simulink model "smm_with_grf_tilting_2d"  (R2014b)
settings: Solver=FixedStepDiscrete  StartTime=0.0  StopTime=inf  FixedStep=sample_time  RelTol=1e-3
undefined symbols (not defined in the file or in its folder): A_lpf_dtau, A_lpf_leg_spring, alpha_apex, alpha_max, alpha_min, B1_lpf_dtau, B1_lpf_leg_spring, B2_lpf_dtau, B2_lpf_leg_spring, boom_mount_angle, boom_pelvis_offset_angle, c_energy, contact_threshold, control_start_time, d_y_boom_com_offset, d_y_boom_hip_offset, d_y_com, desired_torso_angle, dx_avg_desired, enable_torso_wave, fcut_contact, ff_energy_l, ff_energy_r, g, g_reduced, h_boom, HIP_MTR_MAX_CONT_TORQUE, i_robot, initial_com_height, initial_dx, j_leg, j_motor, j_rotor, j_segments, k0_virtual, k_placement, k_sea, kd_lateral, kd_motor, kd_torso, kp_lateral, kp_motor, kp_raibert, kp_torso, l0_leg, l0_min_flight_time, l0_virtual, l0_virtual_raibert, l_boom_projected, l_max, l_retract_delta, l_retract_swing_max, l_retract_swing_min, l_seg, l_yaw_center_to_pelvis, lambda1, lambda2, lateral_offset, lateral_target_angle_left, lateral_target_angle_right ... (+40)
libraries: simulink x24, slrtlib x4, simulink_extras x2
(part 4 of 4)

== matlab function smm_with_grf_tilting_2d/Control/Behavior Control/Secondary Leg Behavior/Virtual Leg Trajectory Towards Alpha Apex Target ==
  data: start input; t_system input; l_leg output; dl_leg output; ddl_leg output; phi output; dphi output; ddphi output; alpha_apex parameter; theta input; l_measured input; dl_measured input; phi_measured input; dphi_measured input; d_y_com parameter; l0_virtual parameter
%% Create a trajectory between starting position/velocity and some alpha
% The goal is to move the system towards the alpha target at apex.
function [l_leg, dl_leg, ddl_leg, phi, dphi, ddphi] = fcn(start, t_system, alpha_apex, theta, l_measured, dl_measured, phi_measured, dphi_measured, d_y_com, l0_virtual)
    % Should the target be less than apex position? midpoint?
    [l_apex, dl_apex, ~, phi_apex, dphi_apex, ~] = AlphaTargetToVirtualLeg2D(alpha_apex, 0, 0, theta, 0, 0, d_y_com, l0_virtual);
    
    % Force retraction when secondary leg
    l_apex = 0.8;
    dl_apex = 0;
    
    persistent t_start l_start phi_start dl_start dphi_start;
    if isempty(t_start)
        t_start = t_system;
        l_start = l_measured;
        dl_start = dl_measured;
        phi_start = phi_measured;
        dphi_start = dphi_measured;
    end
    if start %|| (t_system - t_start) > 0.030
        t_start = t_system;
        l_start = l_measured;
        dl_start = dl_measured;
        phi_start = phi_measured;
        dphi_start = dphi_measured;
    end
    

    time_to_takeoff = 0.350;  % Overestimate, How to approximate this?
    t = t_system - t_start;
    t = min(time_to_takeoff, t);
    
    % Virtual Leg Length
    [a0, a1, a2, a3] = ThirdOrderTrajectory(l_start, dl_start, l_apex, dl_apex, time_to_takeoff);
    l_leg = a3*t^3 + a2*t^2 + a1*t + a0;
    dl_leg = 3*a3*t^2 + 2*a2*t + a1;
    ddl_leg = 6*a3*t + 2*a2;
    
    % Virtual Leg Angle
    [a0, a1, a2, a3] = ThirdOrderTrajectory(phi_start, dphi_start, phi_apex, dphi_apex, time_to_takeoff);
    phi = a3*t^3 + a2*t^2 + a1*t + a0;
    dphi = 3*a3*t^2 + 2*a2*t + a1;
    ddphi = 6*a3*t + 2*a2;
end

== matlab function smm_with_grf_tilting_2d/Control/Behavior Control/Secondary Leg Behavior/Virtual Leg to Four Bar ==
  data: l_leg input; dl_leg input; ddl_leg input; phi input; dphi input; ddphi input; back output; dback output; ddback output; front output; dfront output; ddfront output
function [back, dback, ddback, front, dfront, ddfront] = VirtualLegToFourBar(l_leg, dl_leg, ddl_leg, phi, dphi, ddphi)
    [back, dback, ddback, front, dfront, ddfront] = VirtualLegToFourBar(l_leg, dl_leg, ddl_leg, phi, dphi, ddphi);
end

== matlab function smm_with_grf_tilting_2d/Control/Behavior Control/Primary Leg Behavior/SMM 01/Primary Swing Phase/Leg Trajectory Generator (Level Ground)/Alpha Target to Leg Length and Leg Angle ==
  data: alpha_v input; dalpha_v input; ddalpha_v input; theta input; dtheta input; l output; dl output; ddl output; phi output; d_y_com parameter; l0_virtual parameter; dphi output; ddphi output
function [l, dl, ddl, phi, dphi, ddphi] = fcn(alpha_v, dalpha_v, ddalpha_v, theta, dtheta, d_y_com, l0_virtual)
    [l, dl, ddl, phi, dphi, ddphi] = AlphaTargetToVirtualLeg2D(alpha_v, dalpha_v, ddalpha_v, theta, dtheta, 0, d_y_com, l0_virtual);
end

== matlab function smm_with_grf_tilting_2d/Control/Behavior Control/Primary Leg Behavior/SMM 01/Primary Swing Phase/Leg Trajectory Generator (Level Ground)/Retracted Leg Trajectory ==
  data: start input; t_system input; t_apex input; l_apex input; dl_apex input; phi_apex input; dphi_apex input; l_measured input; dl_measured input; phi_measured input; l output; dl output; ddl output; phi output; dphi output; ddphi output; dphi_measured input
%% Generates a dynamically feasible trajectory for swinging the virtual leg between two points.
% Constrains to starting/ending positions and velocities.
% Minimizes torque squared
% May want to generate the trajectory in fourbar coordinates instead.
function [l, dl, ddl, phi, dphi, ddphi] = fcn(start, t_system, t_apex, l_apex, dl_apex, phi_apex, dphi_apex, l_measured, dl_measured, phi_measured, dphi_measured)

    persistent t_start l_start phi_start dl_start dphi_start;
    if isempty(t_start) || start
        t_start = t_system;
        l_start = l_measured;
        dl_start = dl_measured;
        phi_start = phi_measured;
        dphi_start = dphi_measured;
    end
    
    t = t_system - t_start;
    time_to_apex = 0.95*2*(t_apex - t_start);
    t = min(time_to_apex, t);

    % Virtual Leg Length
    [a0, a1, a2, a3] = ThirdOrderTrajectory(l_start, dl_start, l_apex, dl_apex, time_to_apex);
    l = a3*t^3 + a2*t^2 + a1*t + a0;
    dl = 3*a3*t^2 + 2*a2*t + a1;
    ddl = 6*a3*t + 2*a2;
    
    % Virtual Leg Angle
    [a0, a1, a2, a3] = ThirdOrderTrajectory(phi_start, dphi_start, phi_apex, dphi_apex, time_to_apex);
    phi = a3*t^3 + a2*t^2 + a1*t + a0;
    dphi = 3*a3*t^2 + 2*a2*t + a1;
    ddphi = 6*a3*t + 2*a2;

end

== matlab function smm_with_grf_tilting_2d/Control/Behavior Control/Primary Leg Behavior/SMM 01/Primary Swing Phase/Avoid Hitting Mechanical Limits1 ==
  data: back_cmd output; front_cmd output; dback_cmd output; dfront_cmd output; ddback_cmd output; ddfront_cmd output; back_desired input; dback_desired input; ddback_desired input; front_desired input; dfront_desired input; ddfront_desired input; min_front_bar_angle parameter; max_front_bar_angle parameter; min_back_bar_angle parameter; max_back_bar_angle parameter
%% Avoid joint limits by ensuring we don't command velocities/accelerations that would push us into them when we are close to them.
function [back_cmd, front_cmd, dback_cmd, dfront_cmd, ddback_cmd, ddfront_cmd] ...
    = AvoidFourbarLimits(back_desired,dback_desired, ddback_desired, ...
          front_desired, dfront_desired, ddfront_desired, ...
          min_front_bar_angle, max_front_bar_angle, min_back_bar_angle, max_back_bar_angle)
    [back_cmd, front_cmd, dback_cmd, dfront_cmd, ddback_cmd, ddfront_cmd] = AvoidFourbarLimits(back_desired,dback_desired, ddback_desired, front_desired, dfront_desired, ddfront_desired, min_front_bar_angle, max_front_bar_angle, min_back_bar_angle, max_back_bar_angle);
end

== matlab function smm_with_grf_tilting_2d/Control/Behavior Control/Primary Secondary Leg Swap/ToggleRightLeftLeg ==
  data: toggle input boolean; right_left output double; previous_right_left input double
function right_left = ToggleRightLeftLeg(toggle, previous_right_left)
    
    if toggle
        right_left = -previous_right_left + 1;
    else
        right_left = previous_right_left;
    end

end

== matlab function smm_with_grf_tilting_2d/Control/Behavior Control/Lateral Control ==
  data: tau_r output size=1; qLateralR input; dqLateralR input; qLateralL input; dqLateralL input; F_leg_R input; F_leg_L input; L_leg_R input; L_leg_L input; lateral_transition_force parameter; lateral_target_angle_right parameter; lateral_target_angle_left parameter; boom_mount_angle parameter; boom_pelvis_offset_angle parameter; l_yaw_center_to_pelvis parameter; m_leg_motor parameter; g parameter; lateral_offset parameter; tau_l output size=1; kp_lateral parameter; kd_lateral parameter; minimum_lateral_angle parameter; maximum_lateral_angle parameter; HIP_MTR_MAX_CONT_TORQUE parameter
function [tau_r, tau_l] = LateralBoomControl(qLateralR, dqLateralR, qLateralL, dqLateralL, F_leg_R, F_leg_L, L_leg_R, L_leg_L, lateral_transition_force, lateral_target_angle_right, lateral_target_angle_left, boom_mount_angle, boom_pelvis_offset_angle, l_yaw_center_to_pelvis, m_leg_motor, g, lateral_offset, kp_lateral, kd_lateral, minimum_lateral_angle, maximum_lateral_angle, HIP_MTR_MAX_CONT_TORQUE)

    gravity_compensation = m_leg_motor*g*lateral_offset;
    if (F_leg_R < lateral_transition_force && F_leg_L < lateral_transition_force), gravity_compensation = 0; end % freefall
    
    % Right Leg
    desired = saturate([lateral_target_angle_right, 0],minimum_lateral_angle,maximum_lateral_angle);
    measured = [qLateralR, dqLateralR];
    tau_r = [kp_lateral, kd_lateral] * (desired-measured)' + gravity_compensation;
    tau_r = max(min(HIP_MTR_MAX_CONT_TORQUE, tau_r),-HIP_MTR_MAX_CONT_TORQUE);
    
    if (F_leg_R >= lateral_transition_force)
        angle = qLateralR - boom_pelvis_offset_angle + boom_mount_angle;
        J =   (L_leg_R - l_yaw_center_to_pelvis*sin(angle)) ./ (L_leg_R.*l_yaw_center_to_pelvis.*cos(angle) - l_yaw_center_to_pelvis*lateral_offset*sin(angle));    
        tau_r = -F_leg_R*(J - lateral_offset) + gravity_compensation;
    end
    
    % Left Leg
    desired = saturate([lateral_target_angle_left, 0],minimum_lateral_angle,maximum_lateral_angle);
    measured = [qLateralL, dqLateralL];
    tau_l = [kp_lateral, kd_lateral] * (desired-measured)' + gravity_compensation;
    tau_l = max(min(HIP_MTR_MAX_CONT_TORQUE, tau_l),-HIP_MTR_MAX_CONT_TORQUE);
    
    if (F_leg_L >= lateral_transition_force)
        angle = qLateralL + boom_pelvis_offset_angle - boom_mount_angle;
        J =  -(L_leg_L + l_yaw_center_to_pelvis*sin(angle)) ./ (L_leg_L.*l_yaw_center_to_pelvis.*cos(angle) - l_yaw_center_to_pelvis*lateral_offset*sin(angle));  
        tau_l = F_leg_L*(J - lateral_offset) + gravity_compensation;  
    end
    
    % Stance
%     if ~escape
%         if ~placement && right_or_left
%             angle = qLateralR - boom_pelvis_offset_angle + boom_mount_angle;
%             J =   (l_leg - l_yaw_center_to_pelvis*sin(angle)) ./ (l_leg.*l_yaw_center_to_pelvis.*cos(angle) - l_yaw_center_to_pelvis*lateral_offset*sin(angle));    
%             tau_r = -F_leg*(J - lateral_offset) + gravity_compensation; % + lateral_offset ???  -F*(J+r) + g       F*(J-r) + g
%         elseif ~placement && ~right_or_left
%             angle = qLateralL + boom_pelvis_offset_angle - boom_mount_angle;
%             J =  -(l_leg + l_yaw_center_to_pelvis*sin(angle)) ./ (l_leg.*l_yaw_center_to_pelvis.*cos(angle) - l_yaw_center_to_pelvis*lateral_offset*sin(angle));  
%             tau_l = F_leg*(J - lateral_offset) + gravity_compensation;
%         end
%     end
end

function [desired_saturated] = saturate(desired, minimum_lateral_angle, maximum_lateral_angle)
    desired_saturated = desired;
    if desired(1) < minimum_lateral_angle
        desired_saturated = [minimum_lateral_angle, 0];
    elseif desired(1) > maximum_lateral_angle
        desired_saturated = [maximum_lateral_angle, 0];    
    end
end

== matlab function smm_with_grf_tilting_2d/Control/Behavior Control/Primary Leg Behavior/Raibert Hopping/Inverse Dynamics Virtual Spring/target_GRF_inverse_dynamics ==
  data: z output; k_virtual input; l_virtual input; theta input; phi input; l_leg input; w input; tau_rotor_f input; tau_rotor_b input; d_y_com parameter; l_virtual_rest input; LEG_MTR_GEAR_RATIO parameter; g parameter; j_leg parameter; j_rotor parameter; i_robot parameter; m_total_real parameter; m_boom parameter; m_leg parameter; GRFx output; GRFy output; kp_torso parameter; kd_torso parameter; desired_torso_angle input; GRF_angle output; max_GRF_angle parameter
%% Inverse dynamics
% Inputs:  gamma, dgamma, theta, dtheta,  GRFx_des, GRFy_des
% Outputs: ddx,   ddy,    ddl,   ddgamma, ddtheta,  tau_sf,  tau_sb
function [z, GRFx, GRFy, GRF_angle]  = fcn(k_virtual, l_virtual, theta, phi, l_leg, w,...
                  tau_rotor_f, tau_rotor_b, ...
                  d_y_com, l_virtual_rest, LEG_MTR_GEAR_RATIO, g,...
                  j_leg, j_rotor, i_robot, ...
                  m_total_real, m_boom, m_leg, ...
                  kp_torso, kd_torso, desired_torso_angle, max_GRF_angle)

              
              
    % Parameters
    m      = m_total_real;    % mass of system + boom
    Il     = j_leg;             % inertia of leg
    Ir     = j_rotor;           % inertia of rotor
    It     = i_robot;           % inertia of system
    d      = d_y_com;             % distance from hip to system COM
    g1     = phi(1)+theta(1);   % global leg angle (after spring)
    dg1    = phi(2)+theta(2);
    th     = theta(1);          % global torso angle   
    dth    = theta(2);
    t_rf   = tau_rotor_f;       % torque applied at front rotor 
    t_rb   = tau_rotor_b;       % torque applied at back rotor
    N      = -LEG_MTR_GEAR_RATIO;
    l      = l_leg(1);          % leg length
    dl     = l_leg(2);
    lv     = l_virtual(1);      % virtual spring length
    dx     = -l*dg1*cos(g1)+dth*cos(th);
    dy     = l*dg1*sin(g1)-dth*sin(th);
    
    
    
    % Target GRFs
    delta_lv = l_virtual_rest -  lv;
    GRF = k_virtual*delta_lv* ...
                        [(d*sin(th)-l*sin(g1))/lv; ...
                         (d*cos(th)-l*cos(g1))/lv];
    GRF_angle = atan2(GRF(2),GRF(1));
                     
                     
                     
    % Trunk posture correction 
    % l_leg cross GRF = I_robot * ddtheta
    F_reg = 1; % prevent division by zero
    ddth_desired = kp_torso*(desired_torso_angle - th) - kd_torso*dth; % PD law
    sine_ratio = It*ddth_desired / (lv*(norm(GRF) + F_reg));
    max_angle = 20*pi/180;
    sine_ratio = min(sin(max_angle), max(-sin(max_angle), sine_ratio));  % saturate rotation angle
    GRF_rotation = asin(sine_ratio);
    GRF_full_angle = GRF_rotation + GRF_angle; % saturate GRF angle
    if GRF_full_angle > (pi-max_GRF_angle)
        GRF_rotation = (pi-max_GRF_angle) - GRF_angle;
    elseif GRF_full_angle < max_GRF_angle
        GRF_rotation = max_GRF_angle - GRF_angle;  
    end
    R = [cos(GRF_rotation)  -sin(GRF_rotation); sin(GRF_rotation) cos(GRF_rotation)];
    GRF_target = R*GRF; % rotate GRF CCW
    GRFx = GRF_target(1);
    GRFy = GRF_target(2);
    GRF_angle = atan2(GRFy,GRFx);
    
    
    
    
    % Stance dynamics (P z = [h; -dJ*dq] + [J zeros(2,2)]^T F)
    %     J  = [1  0  sin(g1)     l*cos(g1)   -d*cos(th);
    %           0  1  cos(g1)    -l*sin(g1)    d*sin(th)];
    %       
    %     dJ = [0  0   dg1*cos(g1)    (-l*dg1*sin(g1)+dl*cos(g1))  d*dth*sin(th);
    %           0  0  -dg1*sin(g1)    (-1*dg1*cos(g1)-dl*sin(g1))  d*dth*cos(th)];
    % 
    %     dq  = [dx  dy  dl  dg1  dth ]';
    %       
    %     M = [m  0   0       0    0; 
    %          0  m   0       0    0;
    %          0  0   m_leg   0    0;   
    %          0  0   0       Il   0;  
    %          0  0   0       0    It];  
    %     
    %     h = [0; -m*g_reduced; 0; 0; (-t_rf-t_rb)];
    % 
    %     S = [ 0         0;
    %           0         0;
    %           1/w      -1/w;
    %           1         1;
    %          -(N-1)/N  -(N-1)/N];
    % 
    %     F = [GRFx GRFy]';
    %     
    %     P = [M              -S;       
    %          J               zeros(2,2)];
    
    % Solving for z:    
    %     ddq = [ddx ddy ddl ddg1 ddth]';
    %     z = [ddq; t_sf; t_sb];
    %     z = P\([h; -dJ*dq] + [J zeros(2,2)]'*F);
    
    z =  [GRFx/m;
         (GRFy - g*m)/m;
        -(Il*d*dg1^2*m*cos(g1 - th) - 2*GRFx*Il*d*sin(th) - 2*Il*d^2*dth^2*m - GRFy*d*l^2*m*cos(th) - GRFx*d*l^2*m*sin(th) - 2*GRFy*Il*d*cos(th) + 2*GRFy*It*N*l*cos(g1) + 2*GRFy*Il*N*d*cos(th) + 2*GRFx*It*N*l*sin(g1) + 2*GRFx*Il*N*d*sin(th) - It*N*dg1^2*l*m + GRFy*d*l^2*m*cos(2*g1 - th) + GRFx*d*l^2*m*sin(2*g1 - th) + 2*Il*d*g*m*cos(th) + Il*d*dg1^2*m*cos(g1 + th) + 2*Il*N*d^2*dth^2*m - It*N*dg1^2*l^2*m - 2*It*N*g*l*m*cos(g1) - 2*Il*N*d*g*m*cos(th) + It*N*dg1^2*l^2*m*cos(2*g1) - Il*N*d*dg1^2*m*cos(g1 + th) - Il*d*dg1^2*l*m*cos(g1 + th) + 4*Il*d*dg1*dl*m*sin(g1 - th) + GRFy*N*d^2*l*m*cos(g1) + GRFy*N*d*l^2*m*cos(th) + GRFx*N*d^2*l*m*sin(g1) + 2*N*d*l*m*t_rb*sin(g1 - th) + 2*N*d*l*m*t_rf*sin(g1 - th) + GRFx*N*d*l^2*m*sin(th) - Il*N*d*dg1^2*m*cos(g1 - th) - GRFy*N*d^2*l*m*cos(g1 - 2*th) + GRFx*N*d^2*l*m*sin(g1 - 2*th) + Il*d*dg1^2*l*m*cos(g1 - th) - It*N*dg1^2*l*m*cos(2*g1) - GRFy*N*d*l^2*m*cos(2*g1 - th) - GRFx*N*d*l^2*m*sin(2*g1 - th) + Il*N*d*dg1^2*l*m*cos(g1 + th) - 4*Il*N*d*dg1*dl*m*sin(g1 - th) - Il*N*d*dg1^2*l*m*cos(g1 - th) + 2*It*N*d*dth^2*l*m*cos(g1 - th))/(2*m*(It*N*l - Il*d*cos(g1 - th) + Il*N*d*cos(g1 - th)));
        -(2*GRFx*It*N*cos(g1) - 2*GRFy*It*N*sin(g1) + GRFx*N*d^2*m*cos(g1 - 2*th) + 4*It*N*dg1*dl*m + GRFy*N*d^2*m*sin(g1 - 2*th) + GRFx*d*l*m*cos(2*g1 - th) - GRFy*d*l*m*sin(2*g1 - th) + It*N*dg1^2*m*sin(2*g1) + 2*It*N*g*m*sin(g1) + GRFx*d*l*m*cos(th) - GRFy*d*l*m*sin(th) + GRFx*N*d^2*m*cos(g1) + 2*N*d*m*t_rb*cos(g1 - th) + 2*N*d*m*t_rf*cos(g1 - th) - GRFy*N*d^2*m*sin(g1) - GRFx*N*d*l*m*cos(th) + GRFy*N*d*l*m*sin(th) - GRFx*N*d*l*m*cos(2*g1 - th) - 2*It*N*d*dth^2*m*sin(g1 - th) + GRFy*N*d*l*m*sin(2*g1 - th) - It*N*dg1^2*l*m*sin(2*g1))/(2*m*(It*N*l - Il*d*cos(g1 - th) + Il*N*d*cos(g1 - th)));
        -(GRFx*Il*cos(g1) - GRFy*Il*sin(g1) - GRFx*Il*N*cos(g1) + (Il*dg1^2*m*sin(2*g1))/2 + GRFy*Il*N*sin(g1) + Il*g*m*sin(g1) + GRFx*l^2*m*cos(g1) - GRFy*l^2*m*sin(g1) + 2*Il*dg1*dl*m + N*l*m*t_rb + N*l*m*t_rf + GRFy*N*l^2*m*sin(g1) - 2*Il*N*dg1*dl*m - Il*d*dth^2*m*sin(g1 - th) - (Il*N*dg1^2*m*sin(2*g1))/2 - (Il*dg1^2*l*m*sin(2*g1))/2 - Il*N*g*m*sin(g1) - GRFx*N*l^2*m*cos(g1) + GRFx*N*d*l*m*cos(th) - GRFy*N*d*l*m*sin(th) + Il*N*d*dth^2*m*sin(g1 - th) + (Il*N*dg1^2*l*m*sin(2*g1))/2)/(m*(It*N*l - Il*d*cos(g1 - th) + Il*N*d*cos(g1 - th)));
        -(2*GRFx*Il*It*N*cos(g1) - 2*GRFy*Il*It*N*sin(g1) - GRFy*Il*d*m*w*cos(th) - 2*GRFy*Il*d*m_leg*w*cos(th) - GRFx*Il*d*m*w*sin(th) - 2*GRFx*Il*d*m_leg*w*sin(th) + GRFx*Il*N*d^2*m*cos(g1) + 2*Il*N*d*m*t_rb*cos(g1 - th) + 2*Il*N*d*m*t_rf*cos(g1 - th) + 2*GRFx*It*N*l^2*m*cos(g1) - GRFy*Il*N*d^2*m*sin(g1) - 2*GRFy*It*N*l^2*m*sin(g1) + GRFx*Il*N*d^2*m*cos(g1 - 2*th) + 4*Il*It*N*dg1*dl*m + GRFy*Il*N*d^2*m*sin(g1 - 2*th) - 2*Il*d^2*dth^2*m*m_leg*w - GRFy*Il*d*m*w*cos(2*g1 - th) - GRFx*Il*d*m*w*sin(2*g1 - th) + Il*It*N*dg1^2*m*sin(2*g1) + 2*Il*It*N*g*m*sin(g1) - GRFx*d*l^2*m*m_leg*w*sin(th) - Il*It*N*dg1^2*l*m*sin(2*g1) + Il*d*dg1^2*m*m_leg*w*cos(g1 - th) + 2*GRFy*It*N*l*m*w*cos(g1) + 2*GRFy*It*N*l*m_leg*w*cos(g1) + GRFy*Il*N*d*m*w*cos(th) + 2*GRFy*Il*N*d*m_leg*w*cos(th) + 2*GRFx*It*N*l*m*w*sin(g1) + 2*GRFx*It*N*l*m_leg*w*sin(g1) + GRFx*Il*N*d*m*w*sin(th) + 2*GRFx*Il*N*d*m_leg*w*sin(th) - It*N*dg1^2*l*m*m_leg*w + GRFy*d*l^2*m*m_leg*w*cos(2*g1 - th) + GRFx*d*l^2*m*m_leg*w*sin(2*g1 - th) + 2*Il*d*g*m*m_leg*w*cos(th) + Il*d*dg1^2*m*m_leg*w*cos(g1 + th) + 2*Il*N*d^2*dth^2*m*m_leg*w - It*N*dg1^2*l^2*m*m_leg*w - 2*Il*It*N*d*dth^2*m*sin(g1 - th) + GRFy*Il*N*d*m*w*cos(2*g1 - th) + GRFx*Il*N*d*m*w*sin(2*g1 - th) - GRFy*d*l^2*m*m_leg*w*cos(th) + It*N*dg1^2*l^2*m*m_leg*w*cos(2*g1) - Il*N*d*dg1^2*m*m_leg*w*cos(g1 + th) - Il*d*dg1^2*l*m*m_leg*w*cos(g1 + th) + 4*Il*d*dg1*dl*m*m_leg*w*sin(g1 - th) + GRFy*N*d^2*l*m*m_leg*w*cos(g1) + GRFy*N*d*l^2*m*m_leg*w*cos(th) + GRFx*N*d^2*l*m*m_leg*w*sin(g1) + 2*N*d*l*m*m_leg*t_rb*w*sin(g1 - th) + 2*N*d*l*m*m_leg*t_rf*w*sin(g1 - th) + GRFx*N*d*l^2*m*m_leg*w*sin(th) - Il*N*d*dg1^2*m*m_leg*w*cos(g1 - th) - GRFy*N*d^2*l*m*m_leg*w*cos(g1 - 2*th) + GRFx*N*d^2*l*m*m_leg*w*sin(g1 - 2*th) + Il*d*dg1^2*l*m*m_leg*w*cos(g1 - th) - It*N*dg1^2*l*m*m_leg*w*cos(2*g1) - GRFy*N*d*l^2*m*m_leg*w*cos(2*g1 - th) - GRFx*N*d*l^2*m*m_leg*w*sin(2*g1 - th) - 2*It*N*g*l*m*m_leg*w*cos(g1) - 2*Il*N*d*g*m*m_leg*w*cos(th) + Il*N*d*dg1^2*l*m*m_leg*w*cos(g1 + th) - 4*Il*N*d*dg1*dl*m*m_leg*w*sin(g1 - th) - Il*N*d*dg1^2*l*m*m_leg*w*cos(g1 - th) + 2*It*N*d*dth^2*l*m*m_leg*w*cos(g1 - th))/(4*m*(It*N*l - Il*d*cos(g1 - th) + Il*N*d*cos(g1 - th)));
         (2*GRFy*Il*It*N*sin(g1) - 2*GRFx*Il*It*N*cos(g1) - GRFy*Il*d*m*w*cos(th) - 2*GRFy*Il*d*m_leg*w*cos(th) - GRFx*Il*d*m*w*sin(th) - 2*GRFx*Il*d*m_leg*w*sin(th) - GRFx*Il*N*d^2*m*cos(g1) - 2*Il*N*d*m*t_rb*cos(g1 - th) - 2*Il*N*d*m*t_rf*cos(g1 - th) - 2*GRFx*It*N*l^2*m*cos(g1) + GRFy*Il*N*d^2*m*sin(g1) + 2*GRFy*It*N*l^2*m*sin(g1) - GRFx*Il*N*d^2*m*cos(g1 - 2*th) - 4*Il*It*N*dg1*dl*m - GRFy*Il*N*d^2*m*sin(g1 - 2*th) - 2*Il*d^2*dth^2*m*m_leg*w - GRFy*Il*d*m*w*cos(2*g1 - th) - GRFx*Il*d*m*w*sin(2*g1 - th) - Il*It*N*dg1^2*m*sin(2*g1) - 2*Il*It*N*g*m*sin(g1) - GRFx*d*l^2*m*m_leg*w*sin(th) + Il*It*N*dg1^2*l*m*sin(2*g1) + Il*d*dg1^2*m*m_leg*w*cos(g1 - th) + 2*GRFy*It*N*l*m*w*cos(g1) + 2*GRFy*It*N*l*m_leg*w*cos(g1) + GRFy*Il*N*d*m*w*cos(th) + 2*GRFy*Il*N*d*m_leg*w*cos(th) + 2*GRFx*It*N*l*m*w*sin(g1) + 2*GRFx*It*N*l*m_leg*w*sin(g1) + GRFx*Il*N*d*m*w*sin(th) + 2*GRFx*Il*N*d*m_leg*w*sin(th) - It*N*dg1^2*l*m*m_leg*w + GRFy*d*l^2*m*m_leg*w*cos(2*g1 - th) + GRFx*d*l^2*m*m_leg*w*sin(2*g1 - th) + 2*Il*d*g*m*m_leg*w*cos(th) + Il*d*dg1^2*m*m_leg*w*cos(g1 + th) + 2*Il*N*d^2*dth^2*m*m_leg*w - It*N*dg1^2*l^2*m*m_leg*w + 2*Il*It*N*d*dth^2*m*sin(g1 - th) + GRFy*Il*N*d*m*w*cos(2*g1 - th) + GRFx*Il*N*d*m*w*sin(2*g1 - th) - GRFy*d*l^2*m*m_leg*w*cos(th) + It*N*dg1^2*l^2*m*m_leg*w*cos(2*g1) - Il*N*d*dg1^2*m*m_leg*w*cos(g1 + th) - Il*d*dg1^2*l*m*m_leg*w*cos(g1 + th) + 4*Il*d*dg1*dl*m*m_leg*w*sin(g1 - th) + GRFy*N*d^2*l*m*m_leg*w*cos(g1) + GRFy*N*d*l^2*m*m_leg*w*cos(th) + GRFx*N*d^2*l*m*m_leg*w*sin(g1) + 2*N*d*l*m*m_leg*t_rb*w*sin(g1 - th) + 2*N*d*l*m*m_leg*t_rf*w*sin(g1 - th) + GRFx*N*d*l^2*m*m_leg*w*sin(th) - Il*N*d*dg1^2*m*m_leg*w*cos(g1 - th) - GRFy*N*d^2*l*m*m_leg*w*cos(g1 - 2*th) + GRFx*N*d^2*l*m*m_leg*w*sin(g1 - 2*th) + Il*d*dg1^2*l*m*m_leg*w*cos(g1 - th) - It*N*dg1^2*l*m*m_leg*w*cos(2*g1) - GRFy*N*d*l^2*m*m_leg*w*cos(2*g1 - th) - GRFx*N*d*l^2*m*m_leg*w*sin(2*g1 - th) - 2*It*N*g*l*m*m_leg*w*cos(g1) - 2*Il*N*d*g*m*m_leg*w*cos(th) + Il*N*d*dg1^2*l*m*m_leg*w*cos(g1 + th) - 4*Il*N*d*dg1*dl*m*m_leg*w*sin(g1 - th) - Il*N*d*dg1^2*l*m*m_leg*w*cos(g1 - th) + 2*It*N*d*dth^2*l*m*m_leg*w*cos(g1 - th))/(4*m*(It*N*l - Il*d*cos(g1 - th) + Il*N*d*cos(g1 - th)))];


end

== matlab function smm_with_grf_tilting_2d/Control/Behavior Control/Primary Leg Behavior/Raibert Hopping/Avoid Hitting Mechanical Limits ==
  data: back_cmd output double; front_cmd output double; dback_cmd output double; dfront_cmd output double; ddback_cmd output double; ddfront_cmd output double; back_desired input; dback_desired input; ddback_desired input; front_desired input; dfront_desired input; ddfront_desired input; min_front_bar_angle parameter; max_front_bar_angle parameter; min_back_bar_angle parameter; max_back_bar_angle parameter
%% Avoid joint limits by ensuring we don't command velocities/accelerations that would push us into them when we are close to them.
function [back_cmd, front_cmd, dback_cmd, dfront_cmd, ddback_cmd, ddfront_cmd] ...
    = AvoidFourbarLimits(back_desired,dback_desired, ddback_desired, ...
          front_desired, dfront_desired, ddfront_desired, ...
          min_front_bar_angle, max_front_bar_angle, min_back_bar_angle, max_back_bar_angle)
    [back_cmd, front_cmd, dback_cmd, dfront_cmd, ddback_cmd, ddfront_cmd] = AvoidFourbarLimits(back_desired,dback_desired, ddback_desired, front_desired, dfront_desired, ddfront_desired, min_front_bar_angle, max_front_bar_angle, min_back_bar_angle, max_back_bar_angle);
end

== matlab function smm_with_grf_tilting_2d/Control/Behavior Control/Primary Leg Behavior/Raibert Hopping/Virtual Leg to Four Bar ==
  data: l_leg input; dl_leg input; ddl_leg input; phi input; dphi input; ddphi input; back output; dback output; ddback output; front output; dfront output; ddfront output
function [back, dback, ddback, front, dfront, ddfront] = VirtualLegToFourBar(l_leg, dl_leg, ddl_leg, phi, dphi, ddphi)
    [back, dback, ddback, front, dfront, ddfront] = VirtualLegToFourBar(l_leg, dl_leg, ddl_leg, phi, dphi, ddphi);
end

== matlab function smm_with_grf_tilting_2d/Control/Behavior Control/Primary Leg Behavior/Raibert Hopping/Leg Extension Trajectory1 ==
  data: back input; front input; l_leg output double
function l_leg  = LegLengthCalculator(back, front)
    l_leg = cos((back-front)/2);
end

== matlab function smm_with_grf_tilting_2d/Control/Behavior Control/Primary Leg Behavior/Raibert Hopping/Leg Extension Trajectory ==
  data: t input double; t_trajectory input double; l_leg_final input double; l_leg_initial input double; l_leg output double; dl_leg output double; ddl_leg output double; max_leg_velocity parameter; max_leg_acceleration parameter; min_leg_extension_time parameter
function [l_leg, dl_leg, ddl_leg] = LegLengthTrajectory(t, t_trajectory, l_leg_final, l_leg_initial, max_leg_velocity, max_leg_acceleration, min_leg_extension_time)
    t_trajectory = max(min_leg_extension_time, t_trajectory);
    [l_leg, dl_leg, ddl_leg] = LegLengthTrajectory(t, l_leg_initial, l_leg_final, t_trajectory, max_leg_velocity, max_leg_acceleration);
end

== matlab function smm_with_grf_tilting_2d/Control/Behavior Control/Secondary Leg Behavior/Mirrored Leg Length Target ==
  data: primary_l_leg input; l_leg output; dl_leg output; primary_dl_leg input; l_retract_swing_min parameter; l_retract_swing_max parameter; ddl_leg output; l_retract_delta parameter
function [l_leg, dl_leg, ddl_leg] = LegLengthTarget(primary_l_leg, primary_dl_leg, l_retract_swing_min, l_retract_swing_max, l_retract_delta)

    l_leg = primary_l_leg - l_retract_delta;
    dl_leg = 0;
    ddl_leg = 0;
    if l_leg > l_retract_swing_min && l_leg < l_retract_swing_max
        dl_leg = primary_dl_leg;
    else
        l_leg = max(min(l_leg, l_retract_swing_max), l_retract_swing_min);
    end

end
